simulink model "CSE_Block_Diagram_SimulinkNo2"  (R2023b)
settings: Solver=VariableStepAuto  StartTime=0.0  StopTime=20  RelTol=1e-3
values from neighbouring files (symbols this model uses):
  G1_den = [1 0 0]    [Block_DiagramNo1.m]    (also in Block_DiagramNo2.m; CSE_Block_DiagramNo2.m)
  G1_num = [0 0 1]    [Block_DiagramNo1.m]    (also in Block_DiagramNo2.m = [0 1]; CSE_Block_DiagramNo2.m = [0 1])
  G2_den = [1 1]    [Block_DiagramNo1.m]    (also in Block_DiagramNo2.m; CSE_Block_DiagramNo2.m)
  G2_num = [0 0 1]    [Block_DiagramNo1.m]    (also in Block_DiagramNo2.m = [0 1]; CSE_Block_DiagramNo2.m = [0 1])
  G3_den = [1 0]    [Block_DiagramNo1.m]    (also in Block_DiagramNo2.m; CSE_Block_DiagramNo2.m)
  G3_num = [0 1]    [Block_DiagramNo1.m]    (also in Block_DiagramNo2.m; CSE_Block_DiagramNo2.m)
  G4_den = [2 0]    [Block_DiagramNo2.m]    (also in CSE_Block_DiagramNo2.m)
  G4_num = [0 1]    [Block_DiagramNo2.m]    (also in CSE_Block_DiagramNo2.m)
  G_den = [4 -8 -4 14 -8 -2 2 6 4 0 0 0 0]    [Block_DiagramNo2.m]    (also in CSE_Block_DiagramNo2.m)
  G_num = [2 -6 4 0 0 0 0 0]    [Block_DiagramNo2.m]    (also in CSE_Block_DiagramNo2.m)
  H1_den = [1 0]    [Block_DiagramNo1.m]    (also in Block_DiagramNo2.m; CSE_Block_DiagramNo2.m)
  H1_num = [0 1]    [Block_DiagramNo1.m]    (also in Block_DiagramNo2.m; CSE_Block_DiagramNo2.m)
  H2_den = [1 -1]    [Block_DiagramNo1.m]    (also in Block_DiagramNo2.m; CSE_Block_DiagramNo2.m)
  H2_num = [0 1]    [Block_DiagramNo1.m]    (also in Block_DiagramNo2.m; CSE_Block_DiagramNo2.m)
  H3_den = [1 -2]    [Block_DiagramNo1.m]    (also in Block_DiagramNo2.m; CSE_Block_DiagramNo2.m)
  H3_num = [0 1]    [Block_DiagramNo1.m]    (also in Block_DiagramNo2.m; CSE_Block_DiagramNo2.m)
settings Model: Creator=Laica  LastModifiedBy=Laica

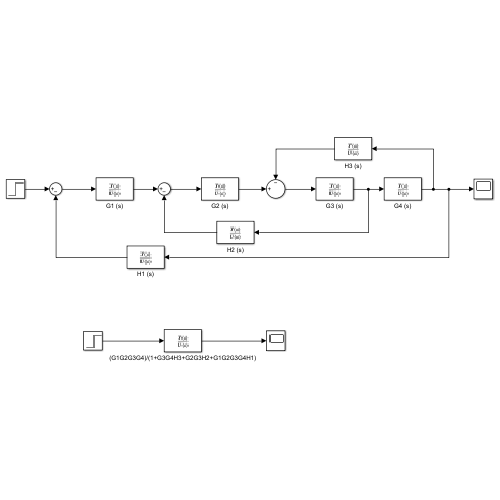
[thumbnail: Simulink's stored preview of the top-level diagram]
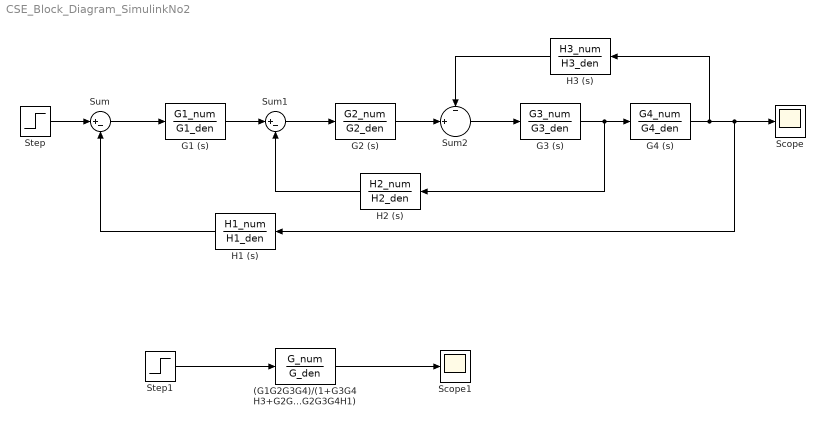
== system CSE_Block_Diagram_SimulinkNo2 ==
  (G1G2G3G4)/(1+G3G4H3+G2G3H2+G1G2G3G4H1) : TransferFcn  Numerator=G_num  Denominator=G_den
  G1 (s) : TransferFcn  Numerator=G1_num  Denominator=G1_den
  G2 (s) : TransferFcn  Numerator=G2_num  Denominator=G2_den
  G3 (s) : TransferFcn  Numerator=G3_num  Denominator=G3_den
  G4 (s) : TransferFcn  Numerator=G4_num  Denominator=G4_den
  H1 (s) : TransferFcn  Numerator=H1_num  Denominator=H1_den
  H2 (s) : TransferFcn  Numerator=H2_num  Denominator=H2_den
  H3 (s) : TransferFcn  Numerator=H3_num  Denominator=H3_den
  Scope : Scope
  Scope1 : Scope
  Step : Step  Time=0  SampleTime=0
  Step1 : Step  Time=0  SampleTime=0
  Sum : Sum  Inputs=|+-
  Sum1 : Sum  Inputs=|+-
  Sum2 : Sum  Inputs=-|+||
  wires:
  Step/1 -> Sum/1
  H1 (s)/1 -> Sum/2
  Sum/1 -> G1 (s)/1
  G1 (s)/1 -> Sum1/1
  H2 (s)/1 -> Sum1/2
  Sum1/1 -> G2 (s)/1
  G2 (s)/1 -> Sum2/2
  H3 (s)/1 -> Sum2/1
  Sum2/1 -> G3 (s)/1
  G3 (s)/1 -> H2 (s)/1, G4 (s)/1
  G4 (s)/1 -> H3 (s)/1, H1 (s)/1, Scope/1
  Step1/1 -> (G1G2G3G4)/(1+G3G4H3+G2G3H2+G1G2G3G4H1)/1
  (G1G2G3G4)/(1+G3G4H3+G2G3H2+G1G2G3G4H1)/1 -> Scope1/1
